simulink model "slabo3"  (R2016b)
settings: Solver=VariableStepAuto  StartTime=0.0  StopTime=10.0  RelTol=1e-3
settings Model: Creator=armenhagopian  LastModifiedBy=armenhagopian

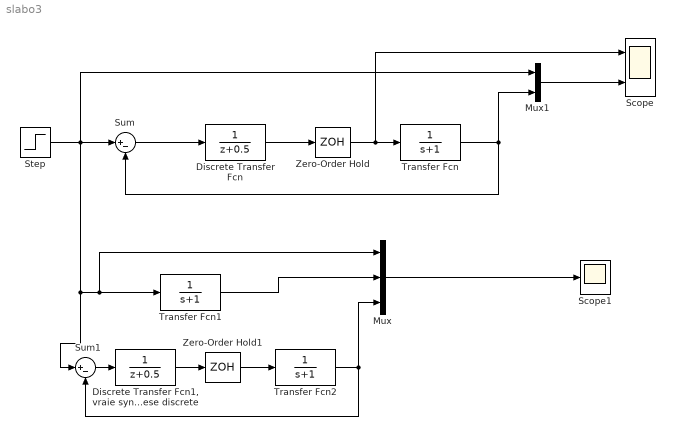
== system slabo3 ==
  Discrete Transfer Fcn : DiscreteTransferFcn
  "Discrete Transfer Fcn1, vraie synthese discrete" : DiscreteTransferFcn
  Mux : Mux  Inputs=3
  Mux1 : Mux  Inputs=2
  Scope : Scope  NumInputPorts=2
  Scope1 : Scope
  Step : Step  SampleTime=0
  Sum : Sum  Inputs=|+-
  Sum1 : Sum  Inputs=|+-
  Transfer Fcn : TransferFcn  Denominator=[1 1]
  Transfer Fcn1 : TransferFcn  Denominator=[1 1]
  Transfer Fcn2 : TransferFcn  Denominator=[1 1]
  Zero-Order Hold : ZeroOrderHold  SampleTime=-1
  Zero-Order Hold1 : ZeroOrderHold  SampleTime=-1
  wires:
  Sum/1 -> Discrete Transfer Fcn/1
  Discrete Transfer Fcn/1 -> Zero-Order Hold/1
  Zero-Order Hold/1 -> Scope/1, Transfer Fcn/1
  Transfer Fcn/1 -> Sum/2, Mux1/2
  Transfer Fcn1/1 -> Mux/2
  Mux/1 -> Scope1/1
  Mux1/1 -> Scope/2
  Step/1 -> Mux/1, Transfer Fcn1/1, Sum1/1, Mux1/1, Sum/1
  "Discrete Transfer Fcn1, vraie synthese discrete"/1 -> Zero-Order Hold1/1
  Zero-Order Hold1/1 -> Transfer Fcn2/1
  Transfer Fcn2/1 -> Sum1/2, Mux/3
  Sum1/1 -> "Discrete Transfer Fcn1, vraie synthese discrete"/1
